simulink model "sm_boom_lift_crawler_flex_boom"  (R2026a)
settings: Solver=ode23t  StopTime=motion.StopTime  MaxStep=2  AbsTol=1e-3  EnableMultiTasking=on
PostLoadFcn:
  | sm_boom_lift_crawler_settest('Tilt test');
  | sm_boom_lift_crawler_generate_boom_ROMs
undefined symbols (not defined in the file or in its folder): motion, X, Y, Z
libraries: sm_lib x22, sm_boom_lift_crawler_lib x11, nesl_utility x4, sm_boom_lift_crawler_lib_boom x1, simulink_extras x1, sm_boom_lift_crawler_lib_inputs x1
Description:
  | Flexible Telescopic Boom
  | 
  | Copyright 2020-2026 The MathWorks, Inc.
settings Model: Creator=smiller  LastModifiedBy=smiller
settings DataIOCC: SignalLoggingName=logsout_sm_boom_lift_crawler
settings SimscapeCC: SimscapeNominalValues="[{\"value\":\"1\",\"unit\":\"A\"},{\"value\":\"nomval_psi\",\"unit\":\"psi\"},{\"value\":\"1\",\"unit\":\"cm^2\"},{\"value\":\"nomval_cmv3_s\",\"unit\":\"cm^3/s\"},{\"value\":\"1\",\"unit\":\"kJ/kg\"},{\"value\":\"1\",\"unit\":\"kW\"},{\"value\":\"1\",\"unit\":\"l\"},{\"value\":\"nomval_N\",\"unit\":\"N\"},{\"value\":\"nomval_Nm\",\"unit\":\"N*m\"},{\"value\":\"1\",\"unit\":\"V\"}]"  SimscapeLogSimulationStatistics=on  SimscapeLogName=simlog_sm_boom_lift_crawler
settings DiagnosticsConfigSet: SimMechanicsConflictingReferenceFrames=none  SimMechanicsRigidlyBoundBlock=none
settings ExplorerConfigSet: InternalSimMechanicsExplorerSettings="<ExplorerConfiguration><canonicalview>default</canonicalview><AnimationSetting><BasePlaybackSpeed>1.0</BasePlaybackSpeed><PlaybackSpeedFactor>1.0</PlaybackSpeedFactor></AnimationSetting><TilePanel><TileInfo><Tiles Columns=\"1\" Count=\"1\" Rows=\"1\"><Column Weight=\"1\"/><Row Weight=\"1\"/><Tile Height=\"1\" Width=\"1\" X=\"0\" Y=\"0\"/></Tiles></TileInfo><SceneInfo><SceneViewer><BGColor><R>1</R><G>1</G><B>1</B></BGColor><Camera><DoPerspective>off</DoPerspective><Position><X>5.10467915842436781</X><Y>18.1042864996443882</Y><Z>4.5660595203260872</Z></Position><Center><X>1.96855945035572688</X><Y>11.6490143272960438</Y><Z>2.66445794602553798</Z></Center><Up><X>-0.0788965068652233703</X><Y>-0.246233868492553493</Y><Z>0.965993904334627729</Z></Up><ViewLimDist>1</ViewLimDist><YLim>4.44954211991442961</YLim><XLim>5.39100695133209218</XLim></Camera></SceneViewer></SceneInfo></TilePanel><MechEditorPanel><Cameras/><GfxPanelCameraMap/><VideoCreator><PlaybackSpeedRatio>1.0</PlaybackSpeedRatio><FrameRate>30</FrameRate><VideoFormat>Motion JPEG AVI</VideoFormat><FrameSize>auto</FrameSize></VideoCreator></MechEditorPanel></ExplorerConfiguration>"

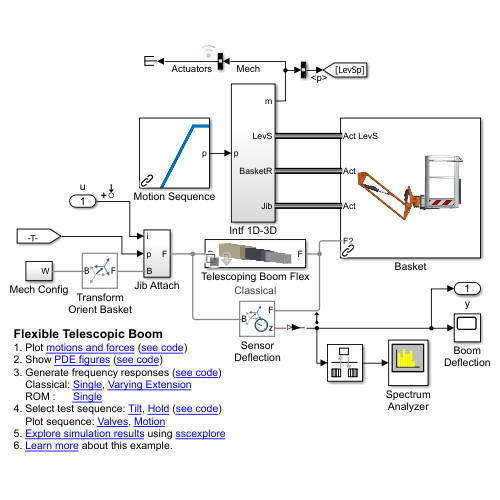
[thumbnail: Simulink's stored preview of the top-level diagram]
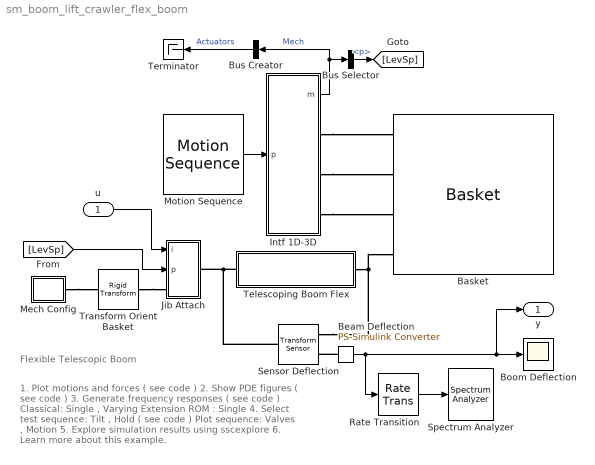
== system sm_boom_lift_crawler_flex_boom ==
  note: Flexible Telescopic Boom
  note: 1. Plot motions and forces ( see code )
      | 2. Show PDE figures ( see code )
      | 3. Generate frequency responses ( see code )
      | Classical: Single , Varying Extension
      | ROM : Single
      | 4. Select test sequence: Tilt , Hold ( see code )
      | Plot sequence: Valves , Motion
      | 5. Explore simulation results using sscexplore
      | 6. Learn more about this example.
  u : Inport
  Basket : sm_boom_lift_crawler_lib_boom/Boom/Basket  SystemSampleTime=-1  VariantActivationTime=update diagram  EmptyChoice=off  PassThrough=off  PassThroughVariantControl=(default)  EmptyChoiceVariantControl=(default)  AllowFlexibleInterface=on  Latency=0  AutoFrameSizeCalculation=off
  Beam Deflection : nesl_utility/PS-Simulink Converter  PhysicalDomain=network_engine_domain  SubClassName=ps_output  LeftPortType=input  RightPortType=output  PseudoPeriodic=off  Frequencies=[]  VectorFormat=1-D array  Unit=m  AffineConversion=off
  Boom Deflection : Scope
      settings: Title=Boom Deflection  ActiveDisplayYMinimum=-1.59347  ActiveDisplayYMaximum=1.14346
  Bus Creator : BusCreator  Inputs=1
  Bus Selector : BusSelector  OutputSignals=LevelS.p
  Intf 1D-3D : Subsystem
  Jib Attach : Subsystem
  Mech Config : Subsystem
  Motion Sequence : sm_boom_lift_crawler_lib_inputs/Motion Sequence  SystemSampleTime=-1  VariantActivationTime=update diagram  EmptyChoice=off  PassThrough=off  PassThroughVariantControl=(default)  EmptyChoiceVariantControl=(default)  AllowFlexibleInterface=on  Latency=0  AutoFrameSizeCalculation=off
  Rate Transition : RateTransition  OutPortSampleTime=0.01
  Sensor Deflection : sm_lib/Frames and Transforms/Transform Sensor  MeasurementFrame=Base  RotationSequence=XYX  SenseAngle=off  SenseAxis=off  SenseQ=off  SenseR=off  SenseRotationSequence=off  SenseOmegaX=off  SenseOmegaY=off  SenseOmegaZ=off  SenseOmega=off  SenseQDot=off  SenseRDot=off  SenseRotationSequenceDot=off  SenseAlphaX=off  SenseAlphaY=off  SenseAlphaZ=off  SenseAlpha=off  SenseQDDot=off  SenseRDDot=off  SenseX=off  SenseY=off  SenseZ=on  SenseXYZ=off  SenseRad=off  SenseAzim=off  SenseDist=off  SenseInc=off  SenseXDot=off  SenseYDot=off  SenseZDot=off  SenseXYZDot=off  SenseRadDot=off  SenseAzimDot=off  SenseDistDot=off  SenseIncDot=off  SenseXDDot=off  SenseYDDot=off  SenseZDDot=off  SenseXYZDDot=off  SenseRadDDot=off  SenseAzimDDot=off  SenseDistDDot=off  SenseIncDDot=off
  Spectrum Analyzer : SpectrumAnalyzer  WindowPosition=[836.2 70.6 641.6 360]  Method=Welch  SampleRate=100  PlotAsTwoSidedSpectrum=off  FrequencyScale=Log  AxesScaling=Manual  Span=10  CenterFrequency=12.5  StartFrequency=0  StopFrequency=50  AveragingMethod=Running  YLimits=[-245.94579788257621544,44.962863886740791486]  AllowFFTLengthLessThanSamplesPerUpdate=on
      settings: OpenAtSimulationStart=off
  Telescoping Boom Flex : Subsystem  Variant=on  VariantControlMode=label  VariantControl=Choice  LabelModeActiveChoice=Classical  mask{popup_flexType=Classical, overlap_pcnt=0.2}
      mask prompts: popup_flexType "Flexible Beam Model"; overlap_pcnt "Amount Retracted (0-0.4)"
      mask init:
      | set_param(gcb,'LabelModeActiveChoice',...
      |     get_param(gcb,'popup_flexType'));
      settings: AttributesFormatString=%<LabelModeActiveChoice>
      mask TypeOptions popup_flexType: Classical | ROM
      mask Callback popup_flexType:
      | maskObj = Simulink.Mask.get(gcb);
      | ovl_h = maskObj.getParameter('overlap_pcnt');
      | if strcmp(get_param(gcb,'popup_flexType'),'Classical')
      |     ovl_h.Visible = 'on';
      | elseif strcmp(get_param(gcb,'popup_flexType'),'ROM')
      |     ovl_h.Visible = 'off';
      | end
      | clear maskObj
      mask Display:
      | blk = sm_boom_lift_activeVariantBlock(gcb);
      | eval(get_param(blk, 'MaskDisplay'));
  Terminator : Terminator
  Transform Orient Basket : sm_lib/Frames and Transforms/Rigid Transform  RotationMethod=StandardAxis  FollAlignAxisA=+X  BaseAlignAxisA=+Y  FollAlignAxisB=+Y  BaseAlignAxisB=+Z  RotationStandardAxis=+Z  RotationAngle=180  RotationAngleUnits=deg  RotationArbitraryAxis=[0 0 1]  RotationSequenceAxes=FollowerAxes  RotationSequence=XYX  RotationSequenceAngles=[0 0 0]  RotationSequenceAnglesUnits=deg  RotationMatrix=[1 0 0; 0 1 0; 0 0 1]  Quaternion=[1 0 0 0]  TranslationMethod=None  TranslationCartesianOffset=[0 0 0]  TranslationCartesianOffsetUnits=m  TranslationStandardAxis=+Z  TranslationStandardOffset=0  TranslationStandardOffsetUnits=m  TranslationROffset=0  TranslationROffsetUnits=m  TranslationThetaOffset=0  TranslationThetaOffsetUnits=deg  TranslationZOffset=0  TranslationZOffsetUnits=m
  y : Outport  VectorParamsAs1DForOutWhenUnconnected=off
  wires:
  Motion Sequence/1 -> Intf 1D-3D/1(p)
  Bus Selector/1 -> [LevSp]  "<p>"
  Intf 1D-3D/1(m) -> Bus Creator/1, Bus Selector/1  "Mech"
  Bus Creator/1 -> Terminator/1  "Actuators"
  Beam Deflection/1 -> Rate Transition/1, y/1, Boom Deflection/1
  Rate Transition/1 -> Spectrum Analyzer/1
  [LevSp] -> Jib Attach/2(p)
  u/1 -> Jib Attach/1(i)
  connections:
  Mech Config/LConn1 -- Transform Orient Basket/LConn1
  Intf 1D-3D/RConn1 -- Basket/RConn1
  Intf 1D-3D/RConn2 -- Basket/RConn2
  Intf 1D-3D/RConn3 -- Basket/RConn3
  Transform Orient Basket/RConn1 -- Jib Attach/LConn1
  Telescoping Boom Flex/LConn1 -- Sensor Deflection/LConn1 -- Jib Attach/RConn1
  Telescoping Boom Flex/RConn1 -- Sensor Deflection/RConn1 -- Basket/RConn4
  Beam Deflection/LConn1 -- Sensor Deflection/RConn2

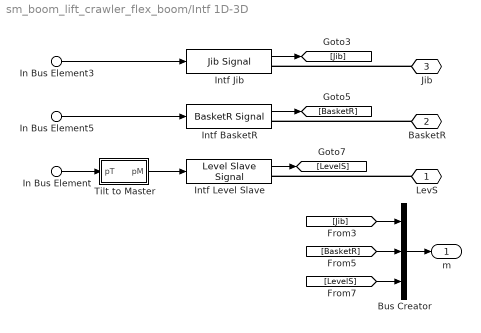
== system sm_boom_lift_crawler_flex_boom/Intf 1D-3D ==
  In Bus Element3 : Inport  PortName=p  Element=Jib
  In Bus Element5 : Inport  PortName=p  Element=BasketR
  In Bus Element : Inport  PortName=p  Element=Tilt
  Bus Creator : BusCreator  Inputs=3
  Intf BasketR : sm_boom_lift_crawler_lib/BasketR Signal  SystemSampleTime=-1  VariantActivationTime=update diagram  EmptyChoice=off  PassThrough=off  PassThroughVariantControl=(default)  EmptyChoiceVariantControl=(default)  AllowFlexibleInterface=on  Latency=0  AutoFrameSizeCalculation=off
  Intf Jib : sm_boom_lift_crawler_lib/Jib Signal  SystemSampleTime=-1  VariantActivationTime=update diagram  EmptyChoice=off  PassThrough=off  PassThroughVariantControl=(default)  EmptyChoiceVariantControl=(default)  AllowFlexibleInterface=on  Latency=0  AutoFrameSizeCalculation=off
  Intf Level Slave : sm_boom_lift_crawler_lib/Level Slave Signal  SystemSampleTime=-1  VariantActivationTime=update diagram  EmptyChoice=off  PassThrough=off  PassThroughVariantControl=(default)  EmptyChoiceVariantControl=(default)  AllowFlexibleInterface=on  Latency=0  AutoFrameSizeCalculation=off
  Tilt to Master : Subsystem
  LevS : PMIOPort  Side=Right
  BasketR : PMIOPort  Port=2  Side=Right
  Jib : PMIOPort  Port=3  Side=Right
  m : Outport
  wires:
  Intf Level Slave/1 -> [LevelS]
  Intf BasketR/1 -> [BasketR]
  Intf Jib/1 -> [Jib]
  [LevelS] -> Bus Creator/3
  Bus Creator/1 -> m/1
  [Jib] -> Bus Creator/1
  [BasketR] -> Bus Creator/2
  In Bus Element3/1 -> Intf Jib/1
  In Bus Element5/1 -> Intf BasketR/1
  In Bus Element/1 -> Tilt to Master/1(pT)
  Tilt to Master/1(pM) -> Intf Level Slave/1
  connections:
  LevS/RConn1 -- Intf Level Slave/RConn1
  BasketR/RConn1 -- Intf BasketR/RConn1
  Jib/RConn1 -- Intf Jib/RConn1

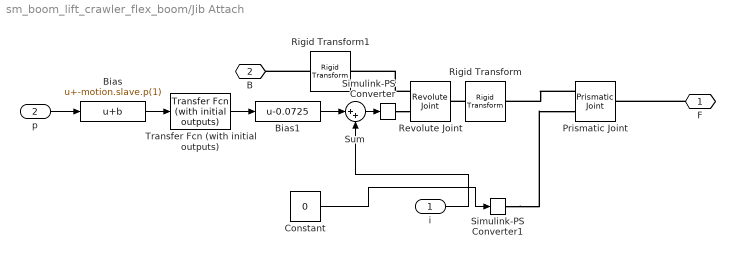
== system sm_boom_lift_crawler_flex_boom/Jib Attach ==
  i : Inport
  p : Inport  Port=2
  Bias : Bias  Bias=-motion.slave.p(1)  SaturateOnIntegerOverflow=off
  Bias1 : Bias  Bias=-0.0725  SaturateOnIntegerOverflow=off
  Constant : Constant  Value=0
  Prismatic Joint : sm_lib/Joints/Prismatic Joint  JointMode=Normal  CompositeWrenchDir=FollowerOnBase  CompositeWrenchFrame=BaseFrame  SenseConstraintForce=off  SenseConstraintTorque=off  SenseTotalForce=off  SenseTotalTorque=off  PositionTargetSpecify=off  PositionTargetPriority=High  PositionTargetValue=0  PositionTargetValueUnits=m  VelocityTargetSpecify=off  VelocityTargetPriority=High  VelocityTargetValue=0  VelocityTargetValueUnits=m/s  EquilibriumPosition=0  EquilibriumPositionUnits=m  SpringStiffness=0  SpringStiffnessUnits=N/m  DampingCoefficient=0  DampingCoefficientUnits=N/(m/s)  LowerLimitSpecify=off  LowerLimitBound=-1  LowerLimitBoundUnits=m  LowerLimitStiffness=1e6  LowerLimitStiffnessUnits=N/m  LowerLimitDamping=1e3  LowerLimitDampingUnits=N/(m/s)  LowerLimitTransitionRegionWidth=1e-4  LowerLimitTransitionRegionWidthUnits=m  UpperLimitSpecify=off  UpperLimitBound=1  UpperLimitBoundUnits=m  UpperLimitStiffness=1e6  UpperLimitStiffnessUnits=N/m  UpperLimitDamping=1e3  UpperLimitDampingUnits=N/(m/s)  UpperLimitTransitionRegionWidth=1e-4  UpperLimitTransitionRegionWidthUnits=m  TorqueActuationMode=ComputedTorque  MotionActuationMode=InputMotion  SensePosition=off  SenseVelocity=off  SenseAcceleration=off  SenseTorqueForce=off  SenseLowerLimitTorqueForce=off  SenseUpperLimitTorqueForce=off
  Revolute Joint : sm_lib/Joints/Revolute Joint  JointMode=Normal  CompositeWrenchDir=FollowerOnBase  CompositeWrenchFrame=BaseFrame  SenseConstraintForce=off  SenseConstraintTorque=off  SenseTotalForce=off  SenseTotalTorque=off  PositionTargetSpecify=on  PositionTargetPriority=High  PositionTargetValue=-0.0725  PositionTargetValueUnits=deg  VelocityTargetSpecify=off  VelocityTargetPriority=High  VelocityTargetValue=0  VelocityTargetValueUnits=deg/s  EquilibriumPosition=0  EquilibriumPositionUnits=deg  SpringStiffness=0  SpringStiffnessUnits=N*m/deg  DampingCoefficient=0  DampingCoefficientUnits=N*m/(deg/s)  LowerLimitSpecify=off  LowerLimitBound=-90  LowerLimitBoundUnits=deg  LowerLimitStiffness=1e4  LowerLimitStiffnessUnits=N*m/deg  LowerLimitDamping=10  LowerLimitDampingUnits=N*m/(deg/s)  LowerLimitTransitionRegionWidth=0.1  LowerLimitTransitionRegionWidthUnits=deg  UpperLimitSpecify=off  UpperLimitBound=90  UpperLimitBoundUnits=deg  UpperLimitStiffness=1e4  UpperLimitStiffnessUnits=N*m/deg  UpperLimitDamping=10  UpperLimitDampingUnits=N*m/(deg/s)  UpperLimitTransitionRegionWidth=0.1  UpperLimitTransitionRegionWidthUnits=deg  TorqueActuationMode=ComputedTorque  MotionActuationMode=InputMotion  SensePosition=off  SenseVelocity=off  SenseAcceleration=off  SenseTorqueForce=off  SenseLowerLimitTorqueForce=off  SenseUpperLimitTorqueForce=off
  Rigid Transform : sm_lib/Frames and Transforms/Rigid Transform  RotationMethod=StandardAxis  FollAlignAxisA=+X  BaseAlignAxisA=+Y  FollAlignAxisB=+Y  BaseAlignAxisB=+Z  RotationStandardAxis=+Y  RotationAngle=90  RotationAngleUnits=deg  RotationArbitraryAxis=[0 0 1]  RotationSequenceAxes=FollowerAxes  RotationSequence=XYX  RotationSequenceAngles=[0 0 0]  RotationSequenceAnglesUnits=deg  RotationMatrix=[1 0 0; 0 1 0; 0 0 1]  Quaternion=[1 0 0 0]  TranslationMethod=None  TranslationCartesianOffset=[0 0 0]  TranslationCartesianOffsetUnits=m  TranslationStandardAxis=+Z  TranslationStandardOffset=0  TranslationStandardOffsetUnits=m  TranslationROffset=0  TranslationROffsetUnits=m  TranslationThetaOffset=0  TranslationThetaOffsetUnits=deg  TranslationZOffset=0  TranslationZOffsetUnits=m
  Rigid Transform1 : sm_lib/Frames and Transforms/Rigid Transform  RotationMethod=StandardAxis  FollAlignAxisA=+X  BaseAlignAxisA=+Y  FollAlignAxisB=+Y  BaseAlignAxisB=+Z  RotationStandardAxis=+Y  RotationAngle=-90  RotationAngleUnits=deg  RotationArbitraryAxis=[0 0 1]  RotationSequenceAxes=FollowerAxes  RotationSequence=XYX  RotationSequenceAngles=[0 0 0]  RotationSequenceAnglesUnits=deg  RotationMatrix=[1 0 0; 0 1 0; 0 0 1]  Quaternion=[1 0 0 0]  TranslationMethod=None  TranslationCartesianOffset=[0 0 0]  TranslationCartesianOffsetUnits=m  TranslationStandardAxis=+Z  TranslationStandardOffset=0  TranslationStandardOffsetUnits=m  TranslationROffset=0  TranslationROffsetUnits=m  TranslationThetaOffset=0  TranslationThetaOffsetUnits=deg  TranslationZOffset=0  TranslationZOffsetUnits=m
  Simulink-PS Converter : nesl_utility/Simulink-PS Converter  PhysicalDomain=network_engine_domain  SubClassName=ps_input  LeftPortType=input  RightPortType=output  PseudoPeriodic=off  Frequencies=[]  NoiseDistribution=none  NoiseParameters=[]  Unit=deg  AffineConversion=off  FilteringAndDerivatives=filter  SimscapeFilterOrder=2  InputFilterTimeConstant=0.001  UdotUserProvided=0
  Simulink-PS Converter1 : nesl_utility/Simulink-PS Converter  PhysicalDomain=network_engine_domain  SubClassName=ps_input  LeftPortType=input  RightPortType=output  PseudoPeriodic=off  Frequencies=[]  NoiseDistribution=none  NoiseParameters=[]  Unit=m  AffineConversion=off  FilteringAndDerivatives=filter  SimscapeFilterOrder=2  InputFilterTimeConstant=0.001  UdotUserProvided=0
  Sum : Sum  Inputs=|++
  Transfer Fcn (with initial outputs) : simulink_extras/Additional Linear/Transfer Fcn (with initial outputs)  N=[400]  D="[0.1  1]"  Y0=0  U0=0
  F : PMIOPort  Side=Right
  B : PMIOPort  Port=2  Side=Left
  wires:
  Transfer Fcn (with initial outputs)/1 -> Bias1/1
  Bias/1 -> Transfer Fcn (with initial outputs)/1
  p/1 -> Bias/1
  Bias1/1 -> Sum/1
  i/1 -> Sum/2
  Sum/1 -> Simulink-PS Converter/1
  Constant/1 -> Simulink-PS Converter1/1
  connections:
  F/RConn1 -- Prismatic Joint/RConn1
  Revolute Joint/LConn1 -- Rigid Transform1/RConn1
  Rigid Transform1/LConn1 -- B/RConn1
  Rigid Transform/LConn1 -- Revolute Joint/RConn1
  Simulink-PS Converter/RConn1 -- Revolute Joint/LConn2
  Prismatic Joint/LConn1 -- Rigid Transform/RConn1
  Simulink-PS Converter1/RConn1 -- Prismatic Joint/LConn2

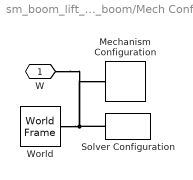
== system sm_boom_lift_crawler_flex_boom/Mech Config ==
  Mechanism Configuration : sm_lib/Utilities/Mechanism Configuration  UniformGravity=Constant  GravityVector=[0 0 -9.80665]  GravityVectorUnits=m/s^2  LinearizationDelta=0.001  JointModeTransitionNonlinearIterations=2
  Solver Configuration : nesl_utility/Solver Configuration  PhysicalDomain=network_engine_domain  SubClassName=solver  LeftPortType=input  RightPortType=generic  Tones=[]  Harmonics=[]  SimulateNoise=off  Profile=off  UseLocalSampling=off  EnableSwitchedLinearOptims=on  FrequencyDomain=off  UseCCode=off  RelTol=0.001  AbsTol=1e-06  MinStep=1e-09  ToWorkspace=off  RevertToSquareIcSolve=off  NumHomotopyIterations=100  PhasorMode=off  PhasorModeNumHarmonics=1  ConsistencySolver=NEWTON_FTOL  CanonicalOrdering=UNORDERED  OptimizeIntermediates=UNOPTIMIZED  IndexReductionMethod=DerivativeReplacement  DoDC=off  ResidualTolerance=1e-9  ConsistencyTolSource=GLOBAL  ConsistencyAbsTol=0.001  ConsistencyRelTol=0.001  ConsistencyTolFactor=0.001  UseLocalSolver=off  LocalSolverChoice=NE_BACKWARD_EULER_ADVANCER  ResolveIndetEquations=on  FunctionEvalNumThread=1  LocalSolverSampleTime=2e-3  DoFixedCost=off  MaxNonlinIter=3  MaxModeIter=2  ComputeImpulses=off  ImpulseIterations=2  LinearAlgebra=auto  LinearAlgebraNumThread=0  EquationFormulation=NE_TIME_EF  DelaysMemoryBudget=1024  AutomaticFiltering=on  FilteringTimeConstant=0.001  PartitionStorageMethod=AS_NEEDED  PartitionMemoryBudget=1024  PartitionMethod=ROBUST  MultibodyUseLocalSolver=off  MultibodyLocalSolverChoice=ODE1  MultibodyLocalSolverSampleTime=0.001
  World : sm_lib/Frames and Transforms/World Frame
  W : PMIOPort  Side=Left
  connections:
  Solver Configuration/RConn1 -- W/RConn1 -- Mechanism Configuration/RConn1 -- World/RConn1

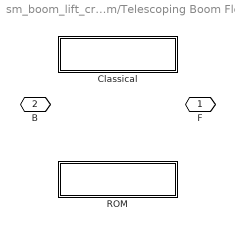
== system sm_boom_lift_crawler_flex_boom/Telescoping Boom Flex ==
  Classical : Subsystem  VariantControl=Classical  mask{overlap=overlap_pcnt, base_w=0.825, mid_w=0.6585, fly_w=0.5335, base_h=1.055, mid_h=0.8745, fly_h=0.757, base_t=0.02082, mid_t=0.02802, fly_t=0.02109, base_l=16.7, mid_l=15.7, fly_l=14.69, base_rho=2700, mid_rho=2700, fly_rho=2700, base_E=70, mid_E=70, fly_E=70, base_v=0.33, mid_v=0.33, fly_v=0.33, base_clr_d=rgb.livery.b.diffuse, mid_clr_d=rgb.metallic.b.diffuse, fly_clr_d=rgb.metallic.e.diffuse, base_clr_s=rgb.livery.b.specular, mid_clr_s=rgb.metallic.b.specular, fly_clr_s=rgb.metallic.e.specular, base_clr_a=rgb.livery.b.ambient, mid_clr_a=rgb.metallic.b.ambient, fly_clr_a=rgb.metallic.e.ambient, base_clr_e=rgb.livery.b.emissive, mid_clr_e=rgb.metallic.b.emissive, fly_clr_e=rgb.metallic.e.emissive, base_clr_h=rgb.livery.b.shininess, mid_clr_h=rgb.metallic.b.shininess, fly_clr_h=rgb.metallic.e.shininess, base_opc=1, mid_opc=1, fly_opc=1}
      mask prompts: overlap "Overlap % (0-1)"
      mask init:
      | overlap_l = overlap*fly_l;
      | 
      | base_extr = [...
      |     base_w/2 base_h/2;
      |     -base_w/2 base_h/2;
      |     -base_w/2 -base_h/2;
      |     base_w/2 -base_h/2;
      |     base_w/2 base_h/2;
      |      (base_w/2-base_t)  (base_h/2-base_t);
      |      (base_w/2-base_t) -(base_h/2-base_t);
      |     -(base_w/2-base_t) -(base_h/2-base_t);
      |     -(base_w/2-base_t)  (base_h/2-base_t);
      |      (base_w/2-base_t)  (base_h/2-base_t);
      |     ];
      mask DialogControl text_base Prompt: Base
      mask DialogControl text_mid Prompt: Mid
      mask DialogControl text_fly Prompt: Fly
      mask DialogControl text_w Prompt: Width (ft)
      mask DialogControl text_h Prompt: Height (ft)
      mask DialogControl text_t Prompt: Thickness (ft)
      mask DialogControl text_l Prompt: Length (ft)
      mask DialogControl text_dens Prompt: Density (kg/m^3)
      mask DialogControl text_E Prompt: Young's Modulus (GPa)
      mask DialogControl text_v Prompt: Poisson's Ratio
      mask DialogControl cont_vis Prompt: Visualization
      mask DialogControl text_base_copy Prompt: Base
      mask DialogControl text_mid_copy Prompt: Mid
      mask DialogControl text_fly_copy Prompt: Fly
      mask DialogControl text_clr_d Prompt: Diffuse Color
      mask DialogControl text_clr_s Prompt: Specular Color
      mask DialogControl text_clr_a Prompt: Ambient Color
      mask DialogControl text_clr_e Prompt: Emissive Color
      mask DialogControl text_clr_h Prompt: Shininess
      mask DialogControl text_opc Prompt: Opacity
      mask Display: image('sm_boom_lift_crawler_flex_telescope_beam.png')
  ROM : Subsystem  VariantControl=ROM  mask{overlap=0.2, base_w=0.825, mid_w=0.6585, fly_w=0.5335, base_h=1.055, mid_h=0.8745, fly_h=0.757, base_t=0.02082, mid_t=0.02802, fly_t=0.02109, base_l=16.7, mid_l=15.7, fly_l=14.69, base_rho=2700, mid_rho=2700, fly_rho=2700, base_E=70, mid_E=70, fly_E=70, base_v=0.33, mid_v=0.33, fly_v=0.33, base_clr_d=rgb.livery.b.diffuse, mid_clr_d=rgb.metallic.b.diffuse, fly_clr_d=rgb.metallic.e.diffuse, base_clr_s=rgb.livery.b.specular, mid_clr_s=rgb.metallic.b.specular, fly_clr_s=rgb.metallic.e.specular, base_clr_a=rgb.livery.b.ambient, mid_clr_a=rgb.metallic.b.ambient, fly_clr_a=rgb.metallic.e.ambient, base_clr_e=rgb.livery.b.emissive, mid_clr_e=rgb.metallic.b.emissive, fly_clr_e=rgb.metallic.e.emissive, base_clr_h=rgb.livery.b.shininess, mid_clr_h=rgb.metallic.b.shininess, fly_clr_h=rgb.metallic.e.shininess, base_opc=0.5, mid_opc=0.5, fly_opc=0.5}
      mask prompts: overlap "Overlap % (0-1)"
      mask init: same as sm_boom_lift_crawler_flex_boom/Telescoping Boom Flex/Classical
      mask DialogControl text_base Prompt: Base
      mask DialogControl text_mid Prompt: Mid
      mask DialogControl text_fly Prompt: Fly
      mask DialogControl text_w Prompt: Width (ft)
      mask DialogControl text_h Prompt: Height (ft)
      mask DialogControl text_t Prompt: Thickness (ft)
      mask DialogControl text_l Prompt: Length (ft)
      mask DialogControl text_dens Prompt: Density (kg/m^3)
      mask DialogControl text_E Prompt: Young's Modulus (GPa)
      mask DialogControl text_v Prompt: Poisson's Ratio
      mask DialogControl cont_vis Prompt: Visualization
      mask DialogControl text_base_copy Prompt: Base
      mask DialogControl text_mid_copy Prompt: Mid
      mask DialogControl text_fly_copy Prompt: Fly
      mask DialogControl text_clr_d Prompt: Diffuse Color
      mask DialogControl text_clr_s Prompt: Specular Color
      mask DialogControl text_clr_a Prompt: Ambient Color
      mask DialogControl text_clr_e Prompt: Emissive Color
      mask DialogControl text_clr_h Prompt: Shininess
      mask DialogControl text_opc Prompt: Opacity
      mask Display: image('sm_boom_lift_crawler_flex_telescope_beam_ROM.png');
  F : PMIOPort  Side=Right
  B : PMIOPort  Port=2  Side=Left

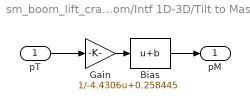
== system sm_boom_lift_crawler_flex_boom/Intf 1D-3D/Tilt to Master ==
  pT : Inport
  Bias : Bias  Bias=0.258445  SaturateOnIntegerOverflow=off
  Gain : Gain  Gain=1/-4.4306
  pM : Outport
  wires:
  Gain/1 -> Bias/1
  pT/1 -> Gain/1
  Bias/1 -> pM/1

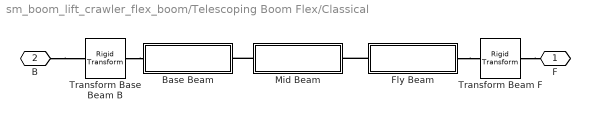
== system sm_boom_lift_crawler_flex_boom/Telescoping Boom Flex/Classical ==
  Base Beam : Subsystem
      mask Display: image('sm_boom_lift_crawler_flex_base.png')
  Fly Beam : Subsystem
      mask Display: image('sm_boom_lift_crawler_flex_fly.png')
  Mid Beam : Subsystem
      mask Display: image('sm_boom_lift_crawler_flex_mid.png')
  Transform Base Beam B : sm_lib/Frames and Transforms/Rigid Transform  RotationMethod=StandardAxis  FollAlignAxisA=+X  BaseAlignAxisA=+Y  FollAlignAxisB=+Y  BaseAlignAxisB=+Z  RotationStandardAxis=+X  RotationAngle=90  RotationAngleUnits=deg  RotationArbitraryAxis=[0 0 1]  RotationSequenceAxes=FollowerAxes  RotationSequence=XYX  RotationSequenceAngles=[0 0 0]  RotationSequenceAnglesUnits=deg  RotationMatrix=[1 0 0; 0 1 0; 0 0 1]  Quaternion=[1 0 0 0]  TranslationMethod=None  TranslationCartesianOffset=[0 0 0]  TranslationCartesianOffsetUnits=m  TranslationStandardAxis=+Z  TranslationStandardOffset=0  TranslationStandardOffsetUnits=m  TranslationROffset=0  TranslationROffsetUnits=m  TranslationThetaOffset=0  TranslationThetaOffsetUnits=deg  TranslationZOffset=0  TranslationZOffsetUnits=m
  Transform Beam F : sm_lib/Frames and Transforms/Rigid Transform  RotationMethod=StandardAxis  FollAlignAxisA=+X  BaseAlignAxisA=+Y  FollAlignAxisB=+Y  BaseAlignAxisB=+Z  RotationStandardAxis=+X  RotationAngle=-90  RotationAngleUnits=deg  RotationArbitraryAxis=[0 0 1]  RotationSequenceAxes=FollowerAxes  RotationSequence=XYX  RotationSequenceAngles=[0 0 0]  RotationSequenceAnglesUnits=deg  RotationMatrix=[1 0 0; 0 1 0; 0 0 1]  Quaternion=[1 0 0 0]  TranslationMethod=None  TranslationCartesianOffset=[0 0 0]  TranslationCartesianOffsetUnits=m  TranslationStandardAxis=+Z  TranslationStandardOffset=0  TranslationStandardOffsetUnits=m  TranslationROffset=0  TranslationROffsetUnits=m  TranslationThetaOffset=0  TranslationThetaOffsetUnits=deg  TranslationZOffset=0  TranslationZOffsetUnits=m
  F : PMIOPort  Side=Right
  B : PMIOPort  Port=2  Side=Left
  connections:
  B/RConn1 -- Transform Base Beam B/LConn1
  Transform Beam F/RConn1 -- F/RConn1
  Transform Base Beam B/RConn1 -- Base Beam/LConn1
  Mid Beam/LConn1 -- Base Beam/RConn1
  Fly Beam/LConn1 -- Mid Beam/RConn1
  Fly Beam/RConn1 -- Transform Beam F/LConn1

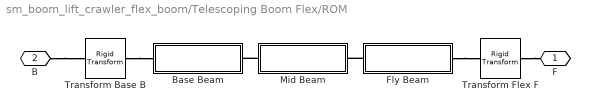
== system sm_boom_lift_crawler_flex_boom/Telescoping Boom Flex/ROM ==
  Base Beam : Subsystem
      mask Display: image('sm_boom_lift_crawler_flex_base_ROM.png')
  Fly Beam : Subsystem
      mask Display: image('sm_boom_lift_crawler_flex_fly_ROM.png')
  Mid Beam : Subsystem
      mask Display: image('sm_boom_lift_crawler_flex_mid_ROM.png')
  Transform Base B : sm_lib/Frames and Transforms/Rigid Transform  RotationMethod=StandardAxis  FollAlignAxisA=+X  BaseAlignAxisA=+Y  FollAlignAxisB=+Y  BaseAlignAxisB=+Z  RotationStandardAxis=+X  RotationAngle=90  RotationAngleUnits=deg  RotationArbitraryAxis=[0 0 1]  RotationSequenceAxes=FollowerAxes  RotationSequence=XYX  RotationSequenceAngles=[0 0 0]  RotationSequenceAnglesUnits=deg  RotationMatrix=[1 0 0; 0 1 0; 0 0 1]  Quaternion=[1 0 0 0]  TranslationMethod=None  TranslationCartesianOffset=[0 0 0]  TranslationCartesianOffsetUnits=m  TranslationStandardAxis=+Z  TranslationStandardOffset=0  TranslationStandardOffsetUnits=m  TranslationROffset=0  TranslationROffsetUnits=m  TranslationThetaOffset=0  TranslationThetaOffsetUnits=deg  TranslationZOffset=0  TranslationZOffsetUnits=m
  Transform Flex F : sm_lib/Frames and Transforms/Rigid Transform  RotationMethod=StandardAxis  FollAlignAxisA=+X  BaseAlignAxisA=+Y  FollAlignAxisB=+Y  BaseAlignAxisB=+Z  RotationStandardAxis=+X  RotationAngle=-90  RotationAngleUnits=deg  RotationArbitraryAxis=[0 0 1]  RotationSequenceAxes=FollowerAxes  RotationSequence=XYX  RotationSequenceAngles=[0 0 0]  RotationSequenceAnglesUnits=deg  RotationMatrix=[1 0 0; 0 1 0; 0 0 1]  Quaternion=[1 0 0 0]  TranslationMethod=None  TranslationCartesianOffset=[0 0 0]  TranslationCartesianOffsetUnits=m  TranslationStandardAxis=+Z  TranslationStandardOffset=0  TranslationStandardOffsetUnits=m  TranslationROffset=0  TranslationROffsetUnits=m  TranslationThetaOffset=0  TranslationThetaOffsetUnits=deg  TranslationZOffset=0  TranslationZOffsetUnits=m
  F : PMIOPort  Side=Right
  B : PMIOPort  Port=2  Side=Left
  connections:
  Fly Beam/RConn1 -- Transform Flex F/LConn1
  Fly Beam/LConn1 -- Mid Beam/RConn1
  Mid Beam/LConn1 -- Base Beam/RConn1
  Transform Base B/RConn1 -- Base Beam/LConn1
  Transform Flex F/RConn1 -- F/RConn1
  B/RConn1 -- Transform Base B/LConn1

== system sm_boom_lift_crawler_flex_boom/Telescoping Boom Flex/Classical/Base Beam ==
  Base Beam : sm_lib/Body Elements/Flexible Bodies/Beams/Flexible Rectangular Beam  SectionType=Hollow  Width=base_w  WidthUnits=ft  Height=base_h  HeightUnits=ft  Thickness=base_t  ThicknessUnits=ft  Length=base_l-overlap_l  LengthUnits=ft  StiffnessAndInertiaType=CalculateFromGeometry  Density=base_rho  DensityUnits=kg/m^3  ModuliType=YoungsPoissons  YoungsModulus=base_E  YoungsModulusUnits=GPa  PoissonsRatio=base_v  ShearModulus=26  ShearModulusUnits=GPa  GeometricCentroid=[0 0]  GeometricCentroidUnits=m  BendingCentroid=[0 0]  BendingCentroidUnits=m  ShearCenter=[0 0]  ShearCenterUnits=m  AxialRigidity=1  AxialRigidityUnits=Pa*m^2  FlexuralRigidity=[1 1]  FlexuralRigidityUnits=Pa*m^4  CrossFlexuralRigidity=0  CrossFlexuralRigidityUnits=Pa*m^4  TorsionalRigidity=1  TorsionalRigidityUnits=Pa*m^4  CenterOfMass=[0 0]  CenterOfMassUnits=m  MassPerUnitLength=1  MassPerUnitLengthUnits=kg/m  MassMomentOfInertiaDensity=[1 1]  MassMomentOfInertiaDensityUnits=kg*m  MassProductOfInertiaDensity=0  MassProductOfInertiaDensityUnits=kg*m  DampingType=Proportional  ProportionalDampingAlpha=0  ProportionalDampingAlphaUnits=1/s  ProportionalDampingBeta=0.001  ProportionalDampingBetaUnits=s  UniformModalDampingRatio=0.01  NumElements=1  ReferenceConditionsType=LinearizedMeanAxes  DoExposeReferenceFrame=off  ReductionType=None  NumRetainedModes=1  GraphicType=FromGeometry  GraphicVisPropType=AdvancedVisualProperties  GraphicDiffuseColor=base_clr_d  GraphicOpacity=base_opc  GraphicSpecularColor=base_clr_s  GraphicAmbientColor=base_clr_a  GraphicEmissiveColor=base_clr_e  GraphicShininess=base_clr_h  DoExposeZminFrame=on  DoExposeZmaxFrame=on  SerializedFrames=<Frames/>
  Overlap Base Mid : sm_boom_lift_crawler_lib/Beam Rigid Segment  beam_h=base_h  beam_w=base_w  beam_t=base_t  beam_l=overlap_l  beam_rho=base_rho  clr_d=base_clr_d  clr_s=base_clr_s  clr_a=base_clr_a  clr_e=base_clr_e  clr_h=base_clr_h  opc=base_opc
  B : PMIOPort  Side=Left
  F : PMIOPort  Port=2  Side=Right
  connections:
  Overlap Base Mid/LConn1 -- Base Beam/RConn1
  B/RConn1 -- Base Beam/LConn1
  Overlap Base Mid/RConn1 -- F/RConn1

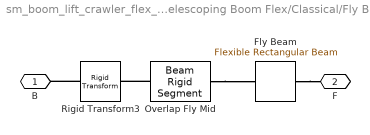
== system sm_boom_lift_crawler_flex_boom/Telescoping Boom Flex/Classical/Fly Beam ==
  Fly Beam : sm_lib/Body Elements/Flexible Bodies/Beams/Flexible Rectangular Beam  SectionType=Hollow  Width=fly_w  WidthUnits=ft  Height=fly_h  HeightUnits=ft  Thickness=fly_t  ThicknessUnits=ft  Length=fly_l-overlap_l  LengthUnits=ft  StiffnessAndInertiaType=CalculateFromGeometry  Density=fly_rho  DensityUnits=kg/m^3  ModuliType=YoungsPoissons  YoungsModulus=fly_E  YoungsModulusUnits=GPa  PoissonsRatio=fly_v  ShearModulus=26  ShearModulusUnits=GPa  GeometricCentroid=[0 0]  GeometricCentroidUnits=m  BendingCentroid=[0 0]  BendingCentroidUnits=m  ShearCenter=[0 0]  ShearCenterUnits=m  AxialRigidity=1  AxialRigidityUnits=Pa*m^2  FlexuralRigidity=[1 1]  FlexuralRigidityUnits=Pa*m^4  CrossFlexuralRigidity=0  CrossFlexuralRigidityUnits=Pa*m^4  TorsionalRigidity=1  TorsionalRigidityUnits=Pa*m^4  CenterOfMass=[0 0]  CenterOfMassUnits=m  MassPerUnitLength=1  MassPerUnitLengthUnits=kg/m  MassMomentOfInertiaDensity=[1 1]  MassMomentOfInertiaDensityUnits=kg*m  MassProductOfInertiaDensity=0  MassProductOfInertiaDensityUnits=kg*m  DampingType=Proportional  ProportionalDampingAlpha=0  ProportionalDampingAlphaUnits=1/s  ProportionalDampingBeta=0.001  ProportionalDampingBetaUnits=s  UniformModalDampingRatio=0.01  NumElements=1  ReferenceConditionsType=LinearizedMeanAxes  DoExposeReferenceFrame=off  ReductionType=None  NumRetainedModes=1  GraphicType=FromGeometry  GraphicVisPropType=AdvancedVisualProperties  GraphicDiffuseColor=fly_clr_d  GraphicOpacity=fly_opc  GraphicSpecularColor=fly_clr_s  GraphicAmbientColor=fly_clr_a  GraphicEmissiveColor=fly_clr_e  GraphicShininess=fly_clr_h  DoExposeZminFrame=on  DoExposeZmaxFrame=on  SerializedFrames=<Frames/>
  Overlap Fly Mid : sm_boom_lift_crawler_lib/Beam Rigid Segment  beam_h=fly_h  beam_w=fly_w  beam_t=fly_t  beam_l=fly_l  beam_rho=fly_rho  clr_d=fly_clr_d  clr_s=fly_clr_s  clr_a=fly_clr_a  clr_e=fly_clr_e  clr_h=fly_clr_h  opc=fly_opc
  Rigid Transform3 : sm_lib/Frames and Transforms/Rigid Transform  RotationMethod=None  FollAlignAxisA=+X  BaseAlignAxisA=+Y  FollAlignAxisB=+Y  BaseAlignAxisB=+Z  RotationStandardAxis=+Z  RotationAngle=0.0  RotationAngleUnits=deg  RotationArbitraryAxis=[0 0 1]  RotationSequenceAxes=FollowerAxes  RotationSequence=XYX  RotationSequenceAngles=[0 0 0]  RotationSequenceAnglesUnits=deg  RotationMatrix=[1 0 0; 0 1 0; 0 0 1]  Quaternion=[1 0 0 0]  TranslationMethod=StandardAxis  TranslationCartesianOffset=[0 0 0]  TranslationCartesianOffsetUnits=ft  TranslationStandardAxis=+Z  TranslationStandardOffset=-overlap_l  TranslationStandardOffsetUnits=ft  TranslationROffset=0  TranslationROffsetUnits=m  TranslationThetaOffset=0  TranslationThetaOffsetUnits=deg  TranslationZOffset=0  TranslationZOffsetUnits=m
  B : PMIOPort  Side=Left
  F : PMIOPort  Port=2  Side=Right
  connections:
  Overlap Fly Mid/RConn1 -- Fly Beam/LConn1
  Rigid Transform3/LConn1 -- B/RConn1
  Overlap Fly Mid/LConn1 -- Rigid Transform3/RConn1
  Fly Beam/RConn1 -- F/RConn1

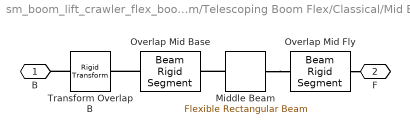
== system sm_boom_lift_crawler_flex_boom/Telescoping Boom Flex/Classical/Mid Beam ==
  "Middle Beam " : sm_lib/Body Elements/Flexible Bodies/Beams/Flexible Rectangular Beam  SectionType=Hollow  Width=mid_w  WidthUnits=ft  Height=mid_h  HeightUnits=ft  Thickness=mid_t  ThicknessUnits=ft  Length=mid_l-2*overlap_l  LengthUnits=ft  StiffnessAndInertiaType=CalculateFromGeometry  Density=mid_rho  DensityUnits=kg/m^3  ModuliType=YoungsPoissons  YoungsModulus=mid_E  YoungsModulusUnits=GPa  PoissonsRatio=mid_v  ShearModulus=26  ShearModulusUnits=GPa  GeometricCentroid=[0 0]  GeometricCentroidUnits=m  BendingCentroid=[0 0]  BendingCentroidUnits=m  ShearCenter=[0 0]  ShearCenterUnits=m  AxialRigidity=1  AxialRigidityUnits=Pa*m^2  FlexuralRigidity=[1 1]  FlexuralRigidityUnits=Pa*m^4  CrossFlexuralRigidity=0  CrossFlexuralRigidityUnits=Pa*m^4  TorsionalRigidity=1  TorsionalRigidityUnits=Pa*m^4  CenterOfMass=[0 0]  CenterOfMassUnits=m  MassPerUnitLength=1  MassPerUnitLengthUnits=kg/m  MassMomentOfInertiaDensity=[1 1]  MassMomentOfInertiaDensityUnits=kg*m  MassProductOfInertiaDensity=0  MassProductOfInertiaDensityUnits=kg*m  DampingType=Proportional  ProportionalDampingAlpha=0  ProportionalDampingAlphaUnits=1/s  ProportionalDampingBeta=0.001  ProportionalDampingBetaUnits=s  UniformModalDampingRatio=0.01  NumElements=1  ReferenceConditionsType=LinearizedMeanAxes  DoExposeReferenceFrame=off  ReductionType=None  NumRetainedModes=1  GraphicType=FromGeometry  GraphicVisPropType=AdvancedVisualProperties  GraphicDiffuseColor=mid_clr_d  GraphicOpacity=mid_opc  GraphicSpecularColor=mid_clr_s  GraphicAmbientColor=mid_clr_a  GraphicEmissiveColor=mid_clr_e  GraphicShininess=mid_clr_h  DoExposeZminFrame=on  DoExposeZmaxFrame=on  SerializedFrames=<Frames/>
  Overlap Mid Base : sm_boom_lift_crawler_lib/Beam Rigid Segment  beam_h=mid_h  beam_w=mid_w  beam_t=mid_t  beam_l=mid_l  beam_rho=mid_rho  clr_d=mid_clr_d  clr_s=mid_clr_s  clr_a=mid_clr_a  clr_e=mid_clr_e  clr_h=mid_clr_h  opc=mid_opc
  Overlap Mid Fly : sm_boom_lift_crawler_lib/Beam Rigid Segment  beam_h=mid_h  beam_w=mid_w  beam_t=mid_t  beam_l=mid_l  beam_rho=mid_rho  clr_d=mid_clr_d  clr_s=mid_clr_s  clr_a=mid_clr_a  clr_e=mid_clr_e  clr_h=mid_clr_h  opc=mid_opc
  Transform Overlap B : sm_lib/Frames and Transforms/Rigid Transform  RotationMethod=None  FollAlignAxisA=+X  BaseAlignAxisA=+Y  FollAlignAxisB=+Y  BaseAlignAxisB=+Z  RotationStandardAxis=+Z  RotationAngle=0.0  RotationAngleUnits=deg  RotationArbitraryAxis=[0 0 1]  RotationSequenceAxes=FollowerAxes  RotationSequence=XYX  RotationSequenceAngles=[0 0 0]  RotationSequenceAnglesUnits=deg  RotationMatrix=[1 0 0; 0 1 0; 0 0 1]  Quaternion=[1 0 0 0]  TranslationMethod=StandardAxis  TranslationCartesianOffset=[0 0 0]  TranslationCartesianOffsetUnits=ft  TranslationStandardAxis=+Z  TranslationStandardOffset=-overlap_l  TranslationStandardOffsetUnits=ft  TranslationROffset=0  TranslationROffsetUnits=m  TranslationThetaOffset=0  TranslationThetaOffsetUnits=deg  TranslationZOffset=0  TranslationZOffsetUnits=m
  B : PMIOPort  Side=Left
  F : PMIOPort  Port=2  Side=Right
  connections:
  Overlap Mid Fly/RConn1 -- F/RConn1
  "Middle Beam "/RConn1 -- Overlap Mid Fly/LConn1
  Overlap Mid Base/LConn1 -- Transform Overlap B/RConn1
  Transform Overlap B/LConn1 -- B/RConn1
  "Middle Beam "/LConn1 -- Overlap Mid Base/RConn1

== system sm_boom_lift_crawler_flex_boom/Telescoping Boom Flex/ROM/Base Beam ==
  Overlap Base Mid : sm_boom_lift_crawler_lib/Beam Rigid Segment  beam_h=base_h  beam_w=base_w  beam_t=base_t  beam_l=overlap_l  beam_rho=base_rho  clr_d=base_clr_d  clr_s=base_clr_s  clr_a=base_clr_a  clr_e=base_clr_e  clr_h=base_clr_h  opc=base_opc
  Reduced Order Flexible Solid : sm_lib/Body Elements/Flexible Bodies/Reduced Order Flexible Solid  UnitSystemType=SI  LengthUnit=m  MassUnit=kg  TimeUnit=s  NumberOfInterfaceFrames=2  InterfaceFrameOrigins=origins_b20  InterfaceFrameOrientations=repmat([1 0 0 0],2,1)  StiffnessMatrix=ROM_b20.K  MassMatrix=ROM_b20.M  DampingType=DampingMatrix  ProportionalDampingAlpha=0  ProportionalDampingBeta=0.001  UniformModalDampingRatio=0.01  DampingMatrix=ROM_b20.C  ReferenceConditionsType=LinearizedMeanAxes  DoExposeReferenceFrame=off  ReductionType=None  NumRetainedModes=1  GraphicType=PartitionedGeometry  GeomFileName=Base_20.STL  GeomUnitType=FromUnitSystem  VisRecursionLimit=3  GraphicVertexCoordinates=[]  GraphicFacetVertexIndices=[]  GraphicReconstructionMatrix=[]  GraphicVisPropType=AdvancedVisualProperties  GraphicDiffuseColor=base_clr_d  GraphicOpacity=1.0  GraphicSpecularColor=base_clr_s  GraphicAmbientColor=base_clr_a  GraphicEmissiveColor=base_clr_e  GraphicShininess=base_clr_h  SenseReducedOrderDOFPosition=off  SenseReducedOrderDOFVelocity=off  SenseReducedOrderDOFAcceleration=off
  B : PMIOPort  Side=Left
  F : PMIOPort  Port=2  Side=Right
  connections:
  Overlap Base Mid/RConn1 -- F/RConn1
  Reduced Order Flexible Solid/LConn1 -- B/RConn1
  Reduced Order Flexible Solid/RConn1 -- Overlap Base Mid/LConn1

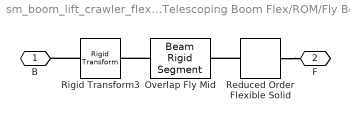
== system sm_boom_lift_crawler_flex_boom/Telescoping Boom Flex/ROM/Fly Beam ==
  Overlap Fly Mid : sm_boom_lift_crawler_lib/Beam Rigid Segment  beam_h=fly_h  beam_w=fly_w  beam_t=fly_t  beam_l=fly_l  beam_rho=fly_rho  clr_d=fly_clr_d  clr_s=fly_clr_s  clr_a=fly_clr_a  clr_e=fly_clr_e  clr_h=fly_clr_h  opc=fly_opc
  Reduced Order Flexible Solid : sm_lib/Body Elements/Flexible Bodies/Reduced Order Flexible Solid  UnitSystemType=SI  LengthUnit=m  MassUnit=kg  TimeUnit=s  NumberOfInterfaceFrames=2  InterfaceFrameOrigins=origins_f20  InterfaceFrameOrientations=repmat([1 0 0 0],2,1)  StiffnessMatrix=ROM_f20.K  MassMatrix=ROM_f20.M  DampingType=DampingMatrix  ProportionalDampingAlpha=0  ProportionalDampingBeta=0.001  UniformModalDampingRatio=0.01  DampingMatrix=ROM_f20.C  ReferenceConditionsType=LinearizedMeanAxes  DoExposeReferenceFrame=off  ReductionType=None  NumRetainedModes=1  GraphicType=PartitionedGeometry  GeomFileName=Fly_20.STL  GeomUnitType=FromUnitSystem  VisRecursionLimit=3  GraphicVertexCoordinates=[]  GraphicFacetVertexIndices=[]  GraphicReconstructionMatrix=[]  GraphicVisPropType=AdvancedVisualProperties  GraphicDiffuseColor=fly_clr_d  GraphicOpacity=1.0  GraphicSpecularColor=fly_clr_s  GraphicAmbientColor=fly_clr_a  GraphicEmissiveColor=fly_clr_e  GraphicShininess=fly_clr_h  SenseReducedOrderDOFPosition=off  SenseReducedOrderDOFVelocity=off  SenseReducedOrderDOFAcceleration=off
  Rigid Transform3 : sm_lib/Frames and Transforms/Rigid Transform  RotationMethod=None  FollAlignAxisA=+X  BaseAlignAxisA=+Y  FollAlignAxisB=+Y  BaseAlignAxisB=+Z  RotationStandardAxis=+Z  RotationAngle=0.0  RotationAngleUnits=deg  RotationArbitraryAxis=[0 0 1]  RotationSequenceAxes=FollowerAxes  RotationSequence=XYX  RotationSequenceAngles=[0 0 0]  RotationSequenceAnglesUnits=deg  RotationMatrix=[1 0 0; 0 1 0; 0 0 1]  Quaternion=[1 0 0 0]  TranslationMethod=StandardAxis  TranslationCartesianOffset=[0 0 0]  TranslationCartesianOffsetUnits=ft  TranslationStandardAxis=+Z  TranslationStandardOffset=-overlap_l  TranslationStandardOffsetUnits=ft  TranslationROffset=0  TranslationROffsetUnits=m  TranslationThetaOffset=0  TranslationThetaOffsetUnits=deg  TranslationZOffset=0  TranslationZOffsetUnits=m
  B : PMIOPort  Side=Left
  F : PMIOPort  Port=2  Side=Right
  connections:
  Reduced Order Flexible Solid/RConn1 -- F/RConn1
  Overlap Fly Mid/LConn1 -- Rigid Transform3/RConn1
  Rigid Transform3/LConn1 -- B/RConn1
  Reduced Order Flexible Solid/LConn1 -- Overlap Fly Mid/RConn1

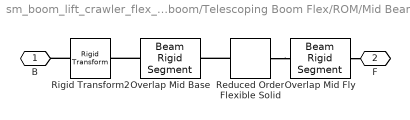
== system sm_boom_lift_crawler_flex_boom/Telescoping Boom Flex/ROM/Mid Beam ==
  Overlap Mid Base : sm_boom_lift_crawler_lib/Beam Rigid Segment  beam_h=mid_h  beam_w=mid_w  beam_t=mid_t  beam_l=mid_l  beam_rho=mid_rho  clr_d=mid_clr_d  clr_s=mid_clr_s  clr_a=mid_clr_a  clr_e=mid_clr_e  clr_h=mid_clr_h  opc=mid_opc
  Overlap Mid Fly : sm_boom_lift_crawler_lib/Beam Rigid Segment  beam_h=mid_h  beam_w=mid_w  beam_t=mid_t  beam_l=mid_l  beam_rho=mid_rho  clr_d=mid_clr_d  clr_s=mid_clr_s  clr_a=mid_clr_a  clr_e=mid_clr_e  clr_h=mid_clr_h  opc=mid_opc
  Reduced Order Flexible Solid : sm_lib/Body Elements/Flexible Bodies/Reduced Order Flexible Solid  UnitSystemType=SI  LengthUnit=m  MassUnit=kg  TimeUnit=s  NumberOfInterfaceFrames=2  InterfaceFrameOrigins=origins_m20  InterfaceFrameOrientations=repmat([1 0 0 0],2,1)  StiffnessMatrix=ROM_m20.K  MassMatrix=ROM_m20.M  DampingType=DampingMatrix  ProportionalDampingAlpha=0  ProportionalDampingBeta=0.001  UniformModalDampingRatio=0.01  DampingMatrix=ROM_m20.C  ReferenceConditionsType=LinearizedMeanAxes  DoExposeReferenceFrame=off  ReductionType=None  NumRetainedModes=1  GraphicType=PartitionedGeometry  GeomFileName=Mid_20.STL  GeomUnitType=FromUnitSystem  VisRecursionLimit=3  GraphicVertexCoordinates=[]  GraphicFacetVertexIndices=[]  GraphicReconstructionMatrix=[]  GraphicVisPropType=AdvancedVisualProperties  GraphicDiffuseColor=mid_clr_d  GraphicOpacity=1.0  GraphicSpecularColor=mid_clr_s  GraphicAmbientColor=mid_clr_a  GraphicEmissiveColor=mid_clr_e  GraphicShininess=mid_clr_h  SenseReducedOrderDOFPosition=off  SenseReducedOrderDOFVelocity=off  SenseReducedOrderDOFAcceleration=off
  Rigid Transform2 : sm_lib/Frames and Transforms/Rigid Transform  RotationMethod=None  FollAlignAxisA=+X  BaseAlignAxisA=+Y  FollAlignAxisB=+Y  BaseAlignAxisB=+Z  RotationStandardAxis=+Z  RotationAngle=0.0  RotationAngleUnits=deg  RotationArbitraryAxis=[0 0 1]  RotationSequenceAxes=FollowerAxes  RotationSequence=XYX  RotationSequenceAngles=[0 0 0]  RotationSequenceAnglesUnits=deg  RotationMatrix=[1 0 0; 0 1 0; 0 0 1]  Quaternion=[1 0 0 0]  TranslationMethod=StandardAxis  TranslationCartesianOffset=[0 0 0]  TranslationCartesianOffsetUnits=ft  TranslationStandardAxis=+Z  TranslationStandardOffset=-overlap_l  TranslationStandardOffsetUnits=ft  TranslationROffset=0  TranslationROffsetUnits=m  TranslationThetaOffset=0  TranslationThetaOffsetUnits=deg  TranslationZOffset=0  TranslationZOffsetUnits=m
  B : PMIOPort  Side=Left
  F : PMIOPort  Port=2  Side=Right
  connections:
  Reduced Order Flexible Solid/LConn1 -- Overlap Mid Base/RConn1
  Rigid Transform2/LConn1 -- B/RConn1
  Overlap Mid Base/LConn1 -- Rigid Transform2/RConn1
  Reduced Order Flexible Solid/RConn1 -- Overlap Mid Fly/LConn1
  Overlap Mid Fly/RConn1 -- F/RConn1
